simulink model "prob1"  (R2018b)
settings: Solver=ode45  StartTime=0.0  StopTime=10.0  RelTol=1e-3  EnableMultiTasking=on
PreLoadFcn:
  | fprintf('*** Loading Puma560 model to workspace\n');
  | mdl_puma560
values from neighbouring files (symbols this model uses):
  p560 = p560.nofriction    [p560_startup_script.m]
undefined symbols (not defined in the file or in its folder): DiscIntNeverNeededParam, qn, transl
libraries: roblocks x5, simulink x1
settings Model: ExtModeTrigMode=oneshot  ExtModeArmWhenConnect=off  Creator=pic  LastModifiedBy=devon
settings DataIOCC: SaveFormat=Array  SignalLoggingSaveFormat=ModelDataLogs
settings OptimizationCC: BlockReduction=off  BooleanDataType=off  ExpressionDepthLimit=2147483647  InitFltsAndDblsToZero=on  LifeSpan=inf
settings DebuggingCC: SaveWithParameterizedLinksMsg=none  UnderspecifiedInitializationDetection=Classic  MergeDetectMultiDrivingBlocksExec=none  SignalResolutionControl=TryResolveAllWithWarning  MultiTaskDSMMsg=warning  MultiTaskCondExecSysMsg=none  FcnCallInpInsideContextMsg=warning  AllowSymbolicDim=off  StateNameClashWarn=warning  SFUnexpectedBacktrackingDiag=warning  SFNoUnconditionalDefaultTransitionDiag=warning  SFExecutionAtInitializationDiag=none
settings HardwareCC: ProdBitPerPointer=32  ProdBitPerSizeT=32  ProdBitPerPtrDiffT=32  ProdLargestAtomicFloat=None  ProdIntDivRoundTo=Undefined  ProdEndianess=Unspecified  ProdWordSize=32  ProdHWDeviceType=32-bit Generic  TargetUnknown=on
settings ModelReferenceCC: PropagateSignalLabelsOutOfModel=off
settings SFSimCC: SimUseLocalCustomCode=off
settings RTWCC: RTWUseLocalCustomCode=off
settings CodeAppCC: StateflowObjectComments=on
settings GRTTargetCC: TargetLangStandard=C89/C90 (ANSI)  ModelReferenceCompliant=off  CompOptLevelCompliant=off  GeneratePreprocessorConditionals=Disable all  CombineOutputUpdateFcns=off  MatFileLogging=off  GRTInterface=on
settings ConfigComp: CovMetricSettings=dw  CovHtmlReporting=on  CovSaveCumulativeToWorkspaceVar=on  CovSaveSingleToWorkspaceVar=on  CovExternalEMLEnable=off

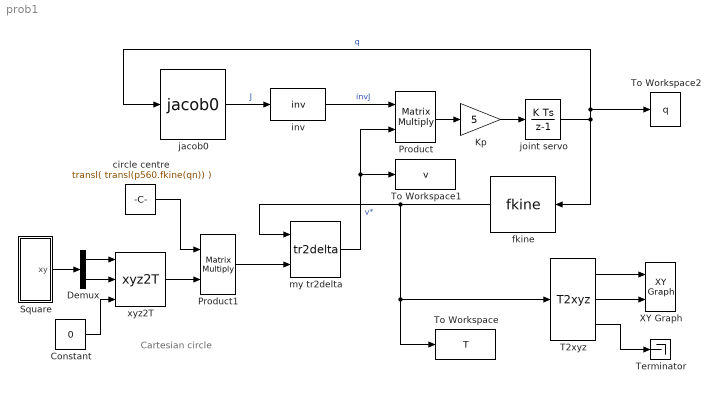
== system prob1 ==
  note: Cartesian circle
  Constant : Constant  Value=0
  Demux : Demux  Outputs=2
  Kp : Gain  Gain=5  SaturateOnIntegerOverflow=on  OutDataTypeStr=Inherit: Same as input  ParamDataTypeStr=Inherit: Same as input
  Product : Product  Multiplication=Matrix(*)  SaturateOnIntegerOverflow=on  RndMeth=Zero  InputSameDT=on  OutDataTypeStr=Inherit: Same as first input
  Product1 : Product  Multiplication=Matrix(*)  SaturateOnIntegerOverflow=on  RndMeth=Zero  InputSameDT=on  OutDataTypeStr=Inherit: Same as first input
  Square : Subsystem  mask{radius=0.05, freq=0.2}
      mask prompts: freq "Frequency (rev/s)"
  T2xyz : roblocks/Toolbox/T2xyz
  Terminator : Terminator
  To Workspace : ToWorkspace  VariableName=T  SampleTime=-1
  To Workspace1 : ToWorkspace  VariableName=v  SampleTime=-1
  To Workspace2 : ToWorkspace  VariableName=q  SampleTime=-1
  XY Graph : simulink/Sinks/XY Graph  xmin=0.5  xmax=0.7  ymin=-0.25  ymax=-0.05  st=-1
  circle centre : Constant  Value=transl( transl(p560.fkine(qn)) )
  fkine : roblocks/Arm/fkine  robot=p560
  inv : MATLABFcn  MATLABFcn=inv  Output1D=off
  "jacob0 " : roblocks/Arm/jacob0   robot=p560
  joint servo : DiscreteIntegrator  InitialCondition=qn'  SampleTime=0.05  ICPrevOutput=DiscIntNeverNeededParam  ICPrevScaledInput=DiscIntNeverNeededParam
  my tr2delta : roblocks/Toolbox/tr2delta
      link override MATLAB Fcn: MATLABFcn=mytr2delta(reshape(u(1:16),4,4), reshape(u(17:32),4,4))
  xyz2T : roblocks/Toolbox/xyz2T
  wires:
  joint servo/1 -> To Workspace2/1, "jacob0 "/1, fkine/1  "q"
  T2xyz/1 -> XY Graph/1
  T2xyz/2 -> XY Graph/2
  my tr2delta/1 -> Product/2, To Workspace1/1  "v*"
  Demux/1 -> xyz2T/1
  "jacob0 "/1 -> inv/1  "J"
  Product/1 -> Kp/1
  inv/1 -> Product/1  "invJ"
  Kp/1 -> joint servo/1
  Demux/2 -> xyz2T/2
  Square/1(xy) -> Demux/1
  Constant/1 -> xyz2T/3
  fkine/1 -> my tr2delta/1, To Workspace/1, T2xyz/1
  xyz2T/1 -> Product1/2
  circle centre/1 -> Product1/1
  T2xyz/3 -> Terminator/1
  Product1/1 -> my tr2delta/2

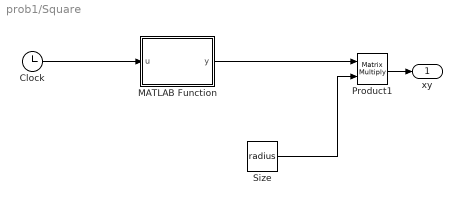
== system prob1/Square ==
  Clock : Clock
  MATLAB Function : MATLAB Function  TreatAsAtomicUnit=on
  Product1 : Product  Multiplication=Matrix(*)  RndMeth=Zero
  Size : Constant  Value=radius
  xy : Outport
  wires:
  Product1/1 -> xy/1
  Size/1 -> Product1/2
  Clock/1 -> MATLAB Function/1(u)
  MATLAB Function/1(y) -> Product1/1

== matlab function prob1/Square/MATLAB Function ==
  data: u input; y output
function y = fcn(u)

y = square(u);
